simulink model "CORDIC_SAP"  (R2021a)
settings: Solver=VariableStepAuto  StartTime=0.0  StopTime=10.0  RelTol=1e-3
undefined symbols (not defined in the file or in its folder): AXI4, Lite
libraries: hdlBasic x278, xbsIndex_r4 x1
(part 1 of 3)
settings Model: Creator=jz118  LastModifiedBy=jz118

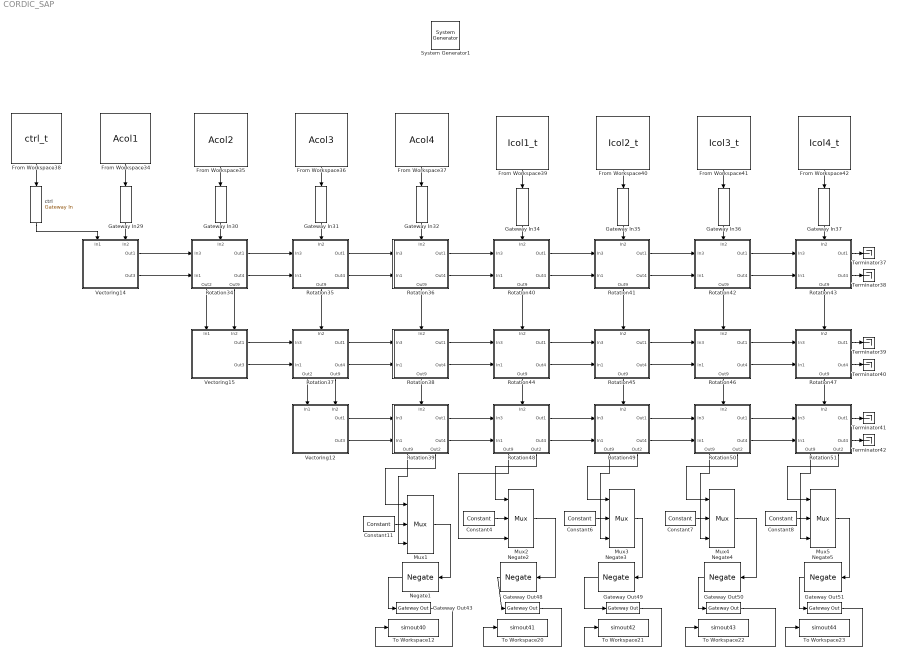
== system CORDIC_SAP ==
  " System Generator1" : xbsIndex_r4/ System Generator  Tag=genX  xilinxfamily=zynq  part=xc7z020  speed=-1  package=clg484  synthesis_tool=Vivado  clock_wrapper=Clock Enables  directory=./netlistAA  proj_type=Vivado  Synth_file=Vivado Synthesis Defaults  Impl_file=Vivado Implementation Defaults  testbench=off  simulink_period=1  sysclk_period=10  dcm_input_clock_period=10  incr_netlist=off  trim_vbits=Everywhere in SubSystem  dbl_ovrd=According to Block Masks  core_generation=According to Block Masks  run_coregen=off  deprecated_control=off  eval_field=0  block_type=sysgen
  Constant{4,6..8,11} (5 alike) : hdlBasic/Constant  const=0  gui_display_data_type=Fixed-point  arith_type=Signed (2's comp)  n_bits=16  bin_pt=13  preci_type=Single  exp_width=8  frac_width=24  explicit_period=off  period=1  XmcBlockStatus=1  maskContainerNames=tabcontainer1  block_type=constant  block_config=sysgen:Constant_config
  From Workspace34 : FromWorkspace  VariableName=Acol1
  From Workspace35 : FromWorkspace  VariableName=Acol2
  From Workspace36 : FromWorkspace  VariableName=Acol3
  From Workspace37 : FromWorkspace  VariableName=Acol4
  From Workspace38 : FromWorkspace  VariableName=ctrl_t
  From Workspace39 : FromWorkspace  VariableName=Icol1_t
  From Workspace40 : FromWorkspace  VariableName=Icol2_t
  From Workspace41 : FromWorkspace  VariableName=Icol3_t
  From Workspace42 : FromWorkspace  VariableName=Icol4_t
  Gateway In29 : hdlBasic/Gateway In  gui_display_data_type=Fixed-point  arith_type=Signed (2's comp)  n_bits=16  bin_pt=13  preci_type=Single  exp_width=8  frac_width=24  rows=1  columns=1  quantization="Round  (unbiased: +/- Inf)"  overflow=Saturate  period=1  UseAsADC=off  ADCChannel='1'  interface=AXI4-Lite  automatic_assignment=on  address_offset=hex2dec('00')  intf_name=''  intf_description='Acol1'  default_value=0  timing_constraint=None  locs_specified=off  LOCs={}  io_standard={}  inherit_from_input=off  hdl_port=on  XmcBlockStatus=1  maskContainerNames=group4  block_type=gatewayin  block_config=sysgen:gateway_in_config  block_width_w=590  block_height_w=620  block_width=640  block_height=850
  Gateway In30 : hdlBasic/Gateway In  gui_display_data_type=Fixed-point  arith_type=Signed (2's comp)  n_bits=16  bin_pt=13  preci_type=Single  exp_width=8  frac_width=24  rows=1  columns=1  quantization="Round  (unbiased: +/- Inf)"  overflow=Saturate  period=1  UseAsADC=off  ADCChannel='1'  interface=AXI4-Lite  automatic_assignment=on  address_offset=hex2dec('00')  intf_name=''  intf_description='Acol2'  default_value=0  timing_constraint=None  locs_specified=off  LOCs={}  io_standard={}  inherit_from_input=off  hdl_port=on  XmcBlockStatus=1  maskContainerNames=group4  block_type=gatewayin  block_config=sysgen:gateway_in_config  block_width_w=590  block_height_w=620  block_width=640  block_height=850
  Gateway In31 : hdlBasic/Gateway In  gui_display_data_type=Fixed-point  arith_type=Signed (2's comp)  n_bits=16  bin_pt=13  preci_type=Single  exp_width=8  frac_width=24  rows=1  columns=1  quantization="Round  (unbiased: +/- Inf)"  overflow=Saturate  period=1  UseAsADC=off  ADCChannel='1'  interface=AXI4-Lite  automatic_assignment=on  address_offset=hex2dec('00')  intf_name=''  intf_description='Acol3'  default_value=0  timing_constraint=None  locs_specified=off  LOCs={}  io_standard={}  inherit_from_input=off  hdl_port=on  XmcBlockStatus=1  maskContainerNames=group4  block_type=gatewayin  block_config=sysgen:gateway_in_config  block_width_w=590  block_height_w=620  block_width=640  block_height=850
  Gateway In32 : hdlBasic/Gateway In  gui_display_data_type=Fixed-point  arith_type=Signed (2's comp)  n_bits=16  bin_pt=13  preci_type=Single  exp_width=8  frac_width=24  rows=1  columns=1  quantization="Round  (unbiased: +/- Inf)"  overflow=Saturate  period=1  UseAsADC=off  ADCChannel='1'  interface=AXI4-Lite  automatic_assignment=on  address_offset=hex2dec('00')  intf_name=''  intf_description='Acol4'  default_value=0  timing_constraint=None  locs_specified=off  LOCs={}  io_standard={}  inherit_from_input=off  hdl_port=on  XmcBlockStatus=1  maskContainerNames=group4  block_type=gatewayin  block_config=sysgen:gateway_in_config  block_width_w=590  block_height_w=620  block_width=640  block_height=850
  Gateway In34 : hdlBasic/Gateway In  gui_display_data_type=Fixed-point  arith_type=Signed (2's comp)  n_bits=16  bin_pt=13  preci_type=Single  exp_width=8  frac_width=24  rows=1  columns=1  quantization="Round  (unbiased: +/- Inf)"  overflow=Saturate  period=1  UseAsADC=off  ADCChannel='1'  interface=AXI4-Lite  automatic_assignment=on  address_offset=hex2dec('00')  intf_name=''  intf_description='Icol1_t'  default_value=0  timing_constraint=None  locs_specified=off  LOCs={}  io_standard={}  inherit_from_input=off  hdl_port=on  XmcBlockStatus=1  maskContainerNames=group4  block_type=gatewayin  block_config=sysgen:gateway_in_config  block_width_w=590  block_height_w=620  block_width=640  block_height=850
  Gateway In35 : hdlBasic/Gateway In  gui_display_data_type=Fixed-point  arith_type=Signed (2's comp)  n_bits=16  bin_pt=13  preci_type=Single  exp_width=8  frac_width=24  rows=1  columns=1  quantization="Round  (unbiased: +/- Inf)"  overflow=Saturate  period=1  UseAsADC=off  ADCChannel='1'  interface=AXI4-Lite  automatic_assignment=on  address_offset=hex2dec('00')  intf_name=''  intf_description='Icol2_t'  default_value=0  timing_constraint=None  locs_specified=off  LOCs={}  io_standard={}  inherit_from_input=off  hdl_port=on  XmcBlockStatus=1  maskContainerNames=group4  block_type=gatewayin  block_config=sysgen:gateway_in_config  block_width_w=590  block_height_w=620  block_width=640  block_height=850
  Gateway In36 : hdlBasic/Gateway In  gui_display_data_type=Fixed-point  arith_type=Signed (2's comp)  n_bits=16  bin_pt=13  preci_type=Single  exp_width=8  frac_width=24  rows=1  columns=1  quantization="Round  (unbiased: +/- Inf)"  overflow=Saturate  period=1  UseAsADC=off  ADCChannel='1'  interface=AXI4-Lite  automatic_assignment=on  address_offset=hex2dec('00')  intf_name=''  intf_description='Icol3_t'  default_value=0  timing_constraint=None  locs_specified=off  LOCs={}  io_standard={}  inherit_from_input=off  hdl_port=on  XmcBlockStatus=1  maskContainerNames=group4  block_type=gatewayin  block_config=sysgen:gateway_in_config  block_width_w=590  block_height_w=620  block_width=640  block_height=850
  Gateway In37 : hdlBasic/Gateway In  gui_display_data_type=Fixed-point  arith_type=Signed (2's comp)  n_bits=16  bin_pt=13  preci_type=Single  exp_width=8  frac_width=24  rows=1  columns=1  quantization="Round  (unbiased: +/- Inf)"  overflow=Saturate  period=1  UseAsADC=off  ADCChannel='1'  interface=AXI4-Lite  automatic_assignment=on  address_offset=hex2dec('00')  intf_name=''  intf_description='Icol4_t'  default_value=0  timing_constraint=None  locs_specified=off  LOCs={}  io_standard={}  inherit_from_input=off  hdl_port=on  XmcBlockStatus=1  maskContainerNames=group4  block_type=gatewayin  block_config=sysgen:gateway_in_config  block_width_w=590  block_height_w=620  block_width=640  block_height=850
  Gateway Out43 : hdlBasic/Gateway Out  inherit_from_input=off  hdl_port=on  rows=1  columns=1  UseAsDAC=off  DACChannel='1'  interface=AXI4-Lite  automatic_assignment=on  address_offset=hex2dec('00')  intf_name=''  intf_description='R_4_4'  timing_constraint=None  locs_specified=off  LOCs={}  io_standard={}  XmcBlockStatus=1  maskContainerNames=group4  block_type=gatewayout  block_config=sysgen:gateway_out_config  block_width_w=590  block_height_w=620  block_width=620  block_height=750
  Gateway Out48 : hdlBasic/Gateway Out  inherit_from_input=off  hdl_port=on  rows=1  columns=1  UseAsDAC=off  DACChannel='1'  interface=AXI4-Lite  automatic_assignment=on  address_offset=hex2dec('00')  intf_name=''  intf_description='Q_4_1'  timing_constraint=None  locs_specified=off  LOCs={}  io_standard={}  XmcBlockStatus=1  maskContainerNames=group4  block_type=gatewayout  block_config=sysgen:gateway_out_config  block_width_w=590  block_height_w=620  block_width=620  block_height=750
  Gateway Out49 : hdlBasic/Gateway Out  inherit_from_input=off  hdl_port=on  rows=1  columns=1  UseAsDAC=off  DACChannel='1'  interface=AXI4-Lite  automatic_assignment=on  address_offset=hex2dec('00')  intf_name=''  intf_description='Q_4_2'  timing_constraint=None  locs_specified=off  LOCs={}  io_standard={}  XmcBlockStatus=1  maskContainerNames=group4  block_type=gatewayout  block_config=sysgen:gateway_out_config  block_width_w=590  block_height_w=620  block_width=620  block_height=750
  Gateway Out50 : hdlBasic/Gateway Out  inherit_from_input=off  hdl_port=on  rows=1  columns=1  UseAsDAC=off  DACChannel='1'  interface=AXI4-Lite  automatic_assignment=on  address_offset=hex2dec('00')  intf_name=''  intf_description='Q_4_3'  timing_constraint=None  locs_specified=off  LOCs={}  io_standard={}  XmcBlockStatus=1  maskContainerNames=group4  block_type=gatewayout  block_config=sysgen:gateway_out_config  block_width_w=590  block_height_w=620  block_width=620  block_height=750
  Gateway Out51 : hdlBasic/Gateway Out  inherit_from_input=off  hdl_port=on  rows=1  columns=1  UseAsDAC=off  DACChannel='1'  interface=AXI4-Lite  automatic_assignment=on  address_offset=hex2dec('00')  intf_name=''  intf_description='Q_4_4'  timing_constraint=None  locs_specified=off  LOCs={}  io_standard={}  XmcBlockStatus=1  maskContainerNames=group4  block_type=gatewayout  block_config=sysgen:gateway_out_config  block_width_w=590  block_height_w=620  block_width=620  block_height=750
  Mux{1..5} (5 alike) : hdlBasic/Mux  inputs=2  en=off  latency=1  precision=Full  arith_type=Unsigned  n_bits=16  bin_pt=14  quantization=Truncate  overflow=Wrap  XmcBlockStatus=1  maskContainerNames=tabcontainer1  block_type=mux  block_config=sysgen:Mux_config
  Negate{1..5} (5 alike) : hdlBasic/Negate  precision=Full  arith_type=Unsigned  n_bits=16  bin_pt=14  quantization=Truncate  overflow=Wrap  en=off  latency=0  XmcBlockStatus=1  maskContainerNames=tabcontainer1  block_type=negate  block_config=sysgen:Negate_config
  Rotation34 : Subsystem
      settings: PortSchema="{\"entries\":[{\"content\":{\"sides\":[{\"content\":{\"connectorIds\":[\"In1\",\"In2\"]},\"type\":\"ConnectorPlacement.EquallySpacedRectSide\",\"uuid\":\"b989bfd3-647b-468d-a24b-67c5817c2fb9\"},{\"content\":{\"connectorIds\":[\"Out1\",\"Out2\"],\"side\":\"RIGHT\"},\"type\":\"ConnectorPlacement.EquallySpacedRectSide\",\"uuid\":\"15839450-c6b9-4b4c-b490-793a0225ad70\"},{\"content\":{\"connectorIds\":[\"In3\"],\"side\":\"TOP\"},\"type\":\"ConnectorPlacement.EquallySpacedRectSide\",\"uuid\":\"69a0ff69-1754-49ce-bc12-3d58954b90b5\"},{\"content\":{\"connectorIds\":[\"Out3\",\"Out4\"],\"side\":\"BOTTOM\"},\"type\":\"ConnectorPlacement.EquallySpacedRectSide\",\"uuid\":\"c7c95c77-bae3-47b7-a54f-9afc9f4e7b60\"}]},\"type\":\"ConnectorPlacement.EquallySpacedConnector\",\"uuid\":\"47487c21-2009-4dc3-9515-f1b42d882620\"}],\"packageUris\":[\"http://schema.mathworks.com/mf0/Connector/R2020b\"],\"version\":\"1.0\"}"
  Rotation35 : Subsystem
      settings: PortSchema="{\"entries\":[{\"content\":{\"sides\":[{\"content\":{\"connectorIds\":[\"In1\",\"In2\"]},\"type\":\"ConnectorPlacement.EquallySpacedRectSide\",\"uuid\":\"b989bfd3-647b-468d-a24b-67c5817c2fb9\"},{\"content\":{\"connectorIds\":[\"Out1\",\"Out2\"],\"side\":\"RIGHT\"},\"type\":\"ConnectorPlacement.EquallySpacedRectSide\",\"uuid\":\"15839450-c6b9-4b4c-b490-793a0225ad70\"},{\"content\":{\"connectorIds\":[\"In3\"],\"side\":\"TOP\"},\"type\":\"ConnectorPlacement.EquallySpacedRectSide\",\"uuid\":\"69a0ff69-1754-49ce-bc12-3d58954b90b5\"},{\"content\":{\"connectorIds\":[\"Out3\"],\"side\":\"BOTTOM\"},\"type\":\"ConnectorPlacement.EquallySpacedRectSide\",\"uuid\":\"c7c95c77-bae3-47b7-a54f-9afc9f4e7b60\"}]},\"type\":\"ConnectorPlacement.EquallySpacedConnector\",\"uuid\":\"47487c21-2009-4dc3-9515-f1b42d882620\"}],\"packageUris\":[\"http://schema.mathworks.com/mf0/Connector/R2020b\"],\"version\":\"1.0\"}"
  Rotation36 : Subsystem
      settings: PortSchema="{\"entries\":[{\"content\":{\"sides\":[{\"content\":{\"connectorIds\":[\"In1\",\"In2\"]},\"type\":\"ConnectorPlacement.EquallySpacedRectSide\",\"uuid\":\"b989bfd3-647b-468d-a24b-67c5817c2fb9\"},{\"content\":{\"connectorIds\":[\"Out1\",\"Out2\"],\"side\":\"RIGHT\"},\"type\":\"ConnectorPlacement.EquallySpacedRectSide\",\"uuid\":\"15839450-c6b9-4b4c-b490-793a0225ad70\"},{\"content\":{\"connectorIds\":[\"In3\"],\"side\":\"TOP\"},\"type\":\"ConnectorPlacement.EquallySpacedRectSide\",\"uuid\":\"69a0ff69-1754-49ce-bc12-3d58954b90b5\"},{\"content\":{\"connectorIds\":[\"Out3\"],\"side\":\"BOTTOM\"},\"type\":\"ConnectorPlacement.EquallySpacedRectSide\",\"uuid\":\"c7c95c77-bae3-47b7-a54f-9afc9f4e7b60\"}]},\"type\":\"ConnectorPlacement.EquallySpacedConnector\",\"uuid\":\"47487c21-2009-4dc3-9515-f1b42d882620\"}],\"packageUris\":[\"http://schema.mathworks.com/mf0/Connector/R2020b\"],\"version\":\"1.0\"}"
  Rotation37 : Subsystem
      settings: PortSchema="{\"entries\":[{\"content\":{\"sides\":[{\"content\":{\"connectorIds\":[\"In1\",\"In2\"]},\"type\":\"ConnectorPlacement.EquallySpacedRectSide\",\"uuid\":\"b989bfd3-647b-468d-a24b-67c5817c2fb9\"},{\"content\":{\"connectorIds\":[\"Out1\",\"Out2\"],\"side\":\"RIGHT\"},\"type\":\"ConnectorPlacement.EquallySpacedRectSide\",\"uuid\":\"15839450-c6b9-4b4c-b490-793a0225ad70\"},{\"content\":{\"connectorIds\":[\"In3\"],\"side\":\"TOP\"},\"type\":\"ConnectorPlacement.EquallySpacedRectSide\",\"uuid\":\"69a0ff69-1754-49ce-bc12-3d58954b90b5\"},{\"content\":{\"connectorIds\":[\"Out3\",\"Out4\"],\"side\":\"BOTTOM\"},\"type\":\"ConnectorPlacement.EquallySpacedRectSide\",\"uuid\":\"c7c95c77-bae3-47b7-a54f-9afc9f4e7b60\"}]},\"type\":\"ConnectorPlacement.EquallySpacedConnector\",\"uuid\":\"47487c21-2009-4dc3-9515-f1b42d882620\"}],\"packageUris\":[\"http://schema.mathworks.com/mf0/Connector/R2020b\"],\"version\":\"1.0\"}"
  Rotation38 : Subsystem
      settings: PortSchema="{\"entries\":[{\"content\":{\"sides\":[{\"content\":{\"connectorIds\":[\"In1\",\"In2\"]},\"type\":\"ConnectorPlacement.EquallySpacedRectSide\",\"uuid\":\"b989bfd3-647b-468d-a24b-67c5817c2fb9\"},{\"content\":{\"connectorIds\":[\"Out1\",\"Out2\"],\"side\":\"RIGHT\"},\"type\":\"ConnectorPlacement.EquallySpacedRectSide\",\"uuid\":\"15839450-c6b9-4b4c-b490-793a0225ad70\"},{\"content\":{\"connectorIds\":[\"In3\"],\"side\":\"TOP\"},\"type\":\"ConnectorPlacement.EquallySpacedRectSide\",\"uuid\":\"69a0ff69-1754-49ce-bc12-3d58954b90b5\"},{\"content\":{\"connectorIds\":[\"Out3\"],\"side\":\"BOTTOM\"},\"type\":\"ConnectorPlacement.EquallySpacedRectSide\",\"uuid\":\"c7c95c77-bae3-47b7-a54f-9afc9f4e7b60\"}]},\"type\":\"ConnectorPlacement.EquallySpacedConnector\",\"uuid\":\"47487c21-2009-4dc3-9515-f1b42d882620\"}],\"packageUris\":[\"http://schema.mathworks.com/mf0/Connector/R2020b\"],\"version\":\"1.0\"}"
  Rotation39 : Subsystem
      settings: PortSchema="{\"entries\":[{\"content\":{\"sides\":[{\"content\":{\"connectorIds\":[\"In1\",\"In2\"]},\"type\":\"ConnectorPlacement.EquallySpacedRectSide\",\"uuid\":\"b989bfd3-647b-468d-a24b-67c5817c2fb9\"},{\"content\":{\"connectorIds\":[\"Out1\",\"Out2\"],\"side\":\"RIGHT\"},\"type\":\"ConnectorPlacement.EquallySpacedRectSide\",\"uuid\":\"15839450-c6b9-4b4c-b490-793a0225ad70\"},{\"content\":{\"connectorIds\":[\"In3\"],\"side\":\"TOP\"},\"type\":\"ConnectorPlacement.EquallySpacedRectSide\",\"uuid\":\"69a0ff69-1754-49ce-bc12-3d58954b90b5\"},{\"content\":{\"connectorIds\":[\"Out3\",\"Out4\"],\"side\":\"BOTTOM\"},\"type\":\"ConnectorPlacement.EquallySpacedRectSide\",\"uuid\":\"c7c95c77-bae3-47b7-a54f-9afc9f4e7b60\"}]},\"type\":\"ConnectorPlacement.EquallySpacedConnector\",\"uuid\":\"47487c21-2009-4dc3-9515-f1b42d882620\"}],\"packageUris\":[\"http://schema.mathworks.com/mf0/Connector/R2020b\"],\"version\":\"1.0\"}"
  Rotation40 : Subsystem
      settings: PortSchema="{\"entries\":[{\"content\":{\"sides\":[{\"content\":{\"connectorIds\":[\"In1\",\"In2\"]},\"type\":\"ConnectorPlacement.EquallySpacedRectSide\",\"uuid\":\"b989bfd3-647b-468d-a24b-67c5817c2fb9\"},{\"content\":{\"connectorIds\":[\"Out1\",\"Out2\"],\"side\":\"RIGHT\"},\"type\":\"ConnectorPlacement.EquallySpacedRectSide\",\"uuid\":\"15839450-c6b9-4b4c-b490-793a0225ad70\"},{\"content\":{\"connectorIds\":[\"In3\"],\"side\":\"TOP\"},\"type\":\"ConnectorPlacement.EquallySpacedRectSide\",\"uuid\":\"69a0ff69-1754-49ce-bc12-3d58954b90b5\"},{\"content\":{\"connectorIds\":[\"Out3\"],\"side\":\"BOTTOM\"},\"type\":\"ConnectorPlacement.EquallySpacedRectSide\",\"uuid\":\"c7c95c77-bae3-47b7-a54f-9afc9f4e7b60\"}]},\"type\":\"ConnectorPlacement.EquallySpacedConnector\",\"uuid\":\"47487c21-2009-4dc3-9515-f1b42d882620\"}],\"packageUris\":[\"http://schema.mathworks.com/mf0/Connector/R2020b\"],\"version\":\"1.0\"}"
  Rotation41 : Subsystem
      settings: PortSchema="{\"entries\":[{\"content\":{\"sides\":[{\"content\":{\"connectorIds\":[\"In1\",\"In2\"]},\"type\":\"ConnectorPlacement.EquallySpacedRectSide\",\"uuid\":\"b989bfd3-647b-468d-a24b-67c5817c2fb9\"},{\"content\":{\"connectorIds\":[\"Out1\",\"Out2\"],\"side\":\"RIGHT\"},\"type\":\"ConnectorPlacement.EquallySpacedRectSide\",\"uuid\":\"15839450-c6b9-4b4c-b490-793a0225ad70\"},{\"content\":{\"connectorIds\":[\"In3\"],\"side\":\"TOP\"},\"type\":\"ConnectorPlacement.EquallySpacedRectSide\",\"uuid\":\"69a0ff69-1754-49ce-bc12-3d58954b90b5\"},{\"content\":{\"connectorIds\":[\"Out3\"],\"side\":\"BOTTOM\"},\"type\":\"ConnectorPlacement.EquallySpacedRectSide\",\"uuid\":\"c7c95c77-bae3-47b7-a54f-9afc9f4e7b60\"}]},\"type\":\"ConnectorPlacement.EquallySpacedConnector\",\"uuid\":\"47487c21-2009-4dc3-9515-f1b42d882620\"}],\"packageUris\":[\"http://schema.mathworks.com/mf0/Connector/R2020b\"],\"version\":\"1.0\"}"
  Rotation42 : Subsystem
      settings: PortSchema="{\"entries\":[{\"content\":{\"sides\":[{\"content\":{\"connectorIds\":[\"In1\",\"In2\"]},\"type\":\"ConnectorPlacement.EquallySpacedRectSide\",\"uuid\":\"b989bfd3-647b-468d-a24b-67c5817c2fb9\"},{\"content\":{\"connectorIds\":[\"Out1\",\"Out2\"],\"side\":\"RIGHT\"},\"type\":\"ConnectorPlacement.EquallySpacedRectSide\",\"uuid\":\"15839450-c6b9-4b4c-b490-793a0225ad70\"},{\"content\":{\"connectorIds\":[\"In3\"],\"side\":\"TOP\"},\"type\":\"ConnectorPlacement.EquallySpacedRectSide\",\"uuid\":\"69a0ff69-1754-49ce-bc12-3d58954b90b5\"},{\"content\":{\"connectorIds\":[\"Out3\"],\"side\":\"BOTTOM\"},\"type\":\"ConnectorPlacement.EquallySpacedRectSide\",\"uuid\":\"c7c95c77-bae3-47b7-a54f-9afc9f4e7b60\"}]},\"type\":\"ConnectorPlacement.EquallySpacedConnector\",\"uuid\":\"47487c21-2009-4dc3-9515-f1b42d882620\"}],\"packageUris\":[\"http://schema.mathworks.com/mf0/Connector/R2020b\"],\"version\":\"1.0\"}"
  Rotation43 : Subsystem
      settings: PortSchema="{\"entries\":[{\"content\":{\"sides\":[{\"content\":{\"connectorIds\":[\"In1\",\"In2\"]},\"type\":\"ConnectorPlacement.EquallySpacedRectSide\",\"uuid\":\"b989bfd3-647b-468d-a24b-67c5817c2fb9\"},{\"content\":{\"connectorIds\":[\"Out1\",\"Out2\"],\"side\":\"RIGHT\"},\"type\":\"ConnectorPlacement.EquallySpacedRectSide\",\"uuid\":\"15839450-c6b9-4b4c-b490-793a0225ad70\"},{\"content\":{\"connectorIds\":[\"In3\"],\"side\":\"TOP\"},\"type\":\"ConnectorPlacement.EquallySpacedRectSide\",\"uuid\":\"69a0ff69-1754-49ce-bc12-3d58954b90b5\"},{\"content\":{\"connectorIds\":[\"Out3\"],\"side\":\"BOTTOM\"},\"type\":\"ConnectorPlacement.EquallySpacedRectSide\",\"uuid\":\"c7c95c77-bae3-47b7-a54f-9afc9f4e7b60\"}]},\"type\":\"ConnectorPlacement.EquallySpacedConnector\",\"uuid\":\"47487c21-2009-4dc3-9515-f1b42d882620\"}],\"packageUris\":[\"http://schema.mathworks.com/mf0/Connector/R2020b\"],\"version\":\"1.0\"}"
  Rotation44 : Subsystem
      settings: PortSchema="{\"entries\":[{\"content\":{\"sides\":[{\"content\":{\"connectorIds\":[\"In1\",\"In2\"]},\"type\":\"ConnectorPlacement.EquallySpacedRectSide\",\"uuid\":\"b989bfd3-647b-468d-a24b-67c5817c2fb9\"},{\"content\":{\"connectorIds\":[\"Out1\",\"Out2\"],\"side\":\"RIGHT\"},\"type\":\"ConnectorPlacement.EquallySpacedRectSide\",\"uuid\":\"15839450-c6b9-4b4c-b490-793a0225ad70\"},{\"content\":{\"connectorIds\":[\"In3\"],\"side\":\"TOP\"},\"type\":\"ConnectorPlacement.EquallySpacedRectSide\",\"uuid\":\"69a0ff69-1754-49ce-bc12-3d58954b90b5\"},{\"content\":{\"connectorIds\":[\"Out3\"],\"side\":\"BOTTOM\"},\"type\":\"ConnectorPlacement.EquallySpacedRectSide\",\"uuid\":\"c7c95c77-bae3-47b7-a54f-9afc9f4e7b60\"}]},\"type\":\"ConnectorPlacement.EquallySpacedConnector\",\"uuid\":\"47487c21-2009-4dc3-9515-f1b42d882620\"}],\"packageUris\":[\"http://schema.mathworks.com/mf0/Connector/R2020b\"],\"version\":\"1.0\"}"
  Rotation45 : Subsystem
      settings: PortSchema="{\"entries\":[{\"content\":{\"sides\":[{\"content\":{\"connectorIds\":[\"In1\",\"In2\"]},\"type\":\"ConnectorPlacement.EquallySpacedRectSide\",\"uuid\":\"b989bfd3-647b-468d-a24b-67c5817c2fb9\"},{\"content\":{\"connectorIds\":[\"Out1\",\"Out2\"],\"side\":\"RIGHT\"},\"type\":\"ConnectorPlacement.EquallySpacedRectSide\",\"uuid\":\"15839450-c6b9-4b4c-b490-793a0225ad70\"},{\"content\":{\"connectorIds\":[\"In3\"],\"side\":\"TOP\"},\"type\":\"ConnectorPlacement.EquallySpacedRectSide\",\"uuid\":\"69a0ff69-1754-49ce-bc12-3d58954b90b5\"},{\"content\":{\"connectorIds\":[\"Out3\"],\"side\":\"BOTTOM\"},\"type\":\"ConnectorPlacement.EquallySpacedRectSide\",\"uuid\":\"c7c95c77-bae3-47b7-a54f-9afc9f4e7b60\"}]},\"type\":\"ConnectorPlacement.EquallySpacedConnector\",\"uuid\":\"47487c21-2009-4dc3-9515-f1b42d882620\"}],\"packageUris\":[\"http://schema.mathworks.com/mf0/Connector/R2020b\"],\"version\":\"1.0\"}"
  Rotation46 : Subsystem
      settings: PortSchema="{\"entries\":[{\"content\":{\"sides\":[{\"content\":{\"connectorIds\":[\"In1\",\"In2\"]},\"type\":\"ConnectorPlacement.EquallySpacedRectSide\",\"uuid\":\"b989bfd3-647b-468d-a24b-67c5817c2fb9\"},{\"content\":{\"connectorIds\":[\"Out1\",\"Out2\"],\"side\":\"RIGHT\"},\"type\":\"ConnectorPlacement.EquallySpacedRectSide\",\"uuid\":\"15839450-c6b9-4b4c-b490-793a0225ad70\"},{\"content\":{\"connectorIds\":[\"In3\"],\"side\":\"TOP\"},\"type\":\"ConnectorPlacement.EquallySpacedRectSide\",\"uuid\":\"69a0ff69-1754-49ce-bc12-3d58954b90b5\"},{\"content\":{\"connectorIds\":[\"Out3\"],\"side\":\"BOTTOM\"},\"type\":\"ConnectorPlacement.EquallySpacedRectSide\",\"uuid\":\"c7c95c77-bae3-47b7-a54f-9afc9f4e7b60\"}]},\"type\":\"ConnectorPlacement.EquallySpacedConnector\",\"uuid\":\"47487c21-2009-4dc3-9515-f1b42d882620\"}],\"packageUris\":[\"http://schema.mathworks.com/mf0/Connector/R2020b\"],\"version\":\"1.0\"}"
  Rotation47 : Subsystem
      settings: PortSchema="{\"entries\":[{\"content\":{\"sides\":[{\"content\":{\"connectorIds\":[\"In1\",\"In2\"]},\"type\":\"ConnectorPlacement.EquallySpacedRectSide\",\"uuid\":\"b989bfd3-647b-468d-a24b-67c5817c2fb9\"},{\"content\":{\"connectorIds\":[\"Out1\",\"Out2\"],\"side\":\"RIGHT\"},\"type\":\"ConnectorPlacement.EquallySpacedRectSide\",\"uuid\":\"15839450-c6b9-4b4c-b490-793a0225ad70\"},{\"content\":{\"connectorIds\":[\"In3\"],\"side\":\"TOP\"},\"type\":\"ConnectorPlacement.EquallySpacedRectSide\",\"uuid\":\"69a0ff69-1754-49ce-bc12-3d58954b90b5\"},{\"content\":{\"connectorIds\":[\"Out3\"],\"side\":\"BOTTOM\"},\"type\":\"ConnectorPlacement.EquallySpacedRectSide\",\"uuid\":\"c7c95c77-bae3-47b7-a54f-9afc9f4e7b60\"}]},\"type\":\"ConnectorPlacement.EquallySpacedConnector\",\"uuid\":\"47487c21-2009-4dc3-9515-f1b42d882620\"}],\"packageUris\":[\"http://schema.mathworks.com/mf0/Connector/R2020b\"],\"version\":\"1.0\"}"
  Rotation48 : Subsystem
      settings: PortSchema="{\"entries\":[{\"content\":{\"sides\":[{\"content\":{\"connectorIds\":[\"In1\",\"In2\"]},\"type\":\"ConnectorPlacement.EquallySpacedRectSide\",\"uuid\":\"b989bfd3-647b-468d-a24b-67c5817c2fb9\"},{\"content\":{\"connectorIds\":[\"Out1\",\"Out2\"],\"side\":\"RIGHT\"},\"type\":\"ConnectorPlacement.EquallySpacedRectSide\",\"uuid\":\"15839450-c6b9-4b4c-b490-793a0225ad70\"},{\"content\":{\"connectorIds\":[\"In3\"],\"side\":\"TOP\"},\"type\":\"ConnectorPlacement.EquallySpacedRectSide\",\"uuid\":\"69a0ff69-1754-49ce-bc12-3d58954b90b5\"},{\"content\":{\"connectorIds\":[\"Out3\",\"Out4\"],\"side\":\"BOTTOM\"},\"type\":\"ConnectorPlacement.EquallySpacedRectSide\",\"uuid\":\"c7c95c77-bae3-47b7-a54f-9afc9f4e7b60\"}]},\"type\":\"ConnectorPlacement.EquallySpacedConnector\",\"uuid\":\"47487c21-2009-4dc3-9515-f1b42d882620\"}],\"packageUris\":[\"http://schema.mathworks.com/mf0/Connector/R2020b\"],\"version\":\"1.0\"}"
  Rotation49 : Subsystem
      settings: PortSchema="{\"entries\":[{\"content\":{\"sides\":[{\"content\":{\"connectorIds\":[\"In1\",\"In2\"]},\"type\":\"ConnectorPlacement.EquallySpacedRectSide\",\"uuid\":\"b989bfd3-647b-468d-a24b-67c5817c2fb9\"},{\"content\":{\"connectorIds\":[\"Out1\",\"Out2\"],\"side\":\"RIGHT\"},\"type\":\"ConnectorPlacement.EquallySpacedRectSide\",\"uuid\":\"15839450-c6b9-4b4c-b490-793a0225ad70\"},{\"content\":{\"connectorIds\":[\"In3\"],\"side\":\"TOP\"},\"type\":\"ConnectorPlacement.EquallySpacedRectSide\",\"uuid\":\"69a0ff69-1754-49ce-bc12-3d58954b90b5\"},{\"content\":{\"connectorIds\":[\"Out3\",\"Out4\"],\"side\":\"BOTTOM\"},\"type\":\"ConnectorPlacement.EquallySpacedRectSide\",\"uuid\":\"c7c95c77-bae3-47b7-a54f-9afc9f4e7b60\"}]},\"type\":\"ConnectorPlacement.EquallySpacedConnector\",\"uuid\":\"47487c21-2009-4dc3-9515-f1b42d882620\"}],\"packageUris\":[\"http://schema.mathworks.com/mf0/Connector/R2020b\"],\"version\":\"1.0\"}"
  Rotation50 : Subsystem
      settings: PortSchema="{\"entries\":[{\"content\":{\"sides\":[{\"content\":{\"connectorIds\":[\"In1\",\"In2\"]},\"type\":\"ConnectorPlacement.EquallySpacedRectSide\",\"uuid\":\"b989bfd3-647b-468d-a24b-67c5817c2fb9\"},{\"content\":{\"connectorIds\":[\"Out1\",\"Out2\"],\"side\":\"RIGHT\"},\"type\":\"ConnectorPlacement.EquallySpacedRectSide\",\"uuid\":\"15839450-c6b9-4b4c-b490-793a0225ad70\"},{\"content\":{\"connectorIds\":[\"In3\"],\"side\":\"TOP\"},\"type\":\"ConnectorPlacement.EquallySpacedRectSide\",\"uuid\":\"69a0ff69-1754-49ce-bc12-3d58954b90b5\"},{\"content\":{\"connectorIds\":[\"Out3\",\"Out4\"],\"side\":\"BOTTOM\"},\"type\":\"ConnectorPlacement.EquallySpacedRectSide\",\"uuid\":\"c7c95c77-bae3-47b7-a54f-9afc9f4e7b60\"}]},\"type\":\"ConnectorPlacement.EquallySpacedConnector\",\"uuid\":\"47487c21-2009-4dc3-9515-f1b42d882620\"}],\"packageUris\":[\"http://schema.mathworks.com/mf0/Connector/R2020b\"],\"version\":\"1.0\"}"
  Rotation51 : Subsystem
      settings: PortSchema="{\"entries\":[{\"content\":{\"sides\":[{\"content\":{\"connectorIds\":[\"In1\",\"In2\"]},\"type\":\"ConnectorPlacement.EquallySpacedRectSide\",\"uuid\":\"b989bfd3-647b-468d-a24b-67c5817c2fb9\"},{\"content\":{\"connectorIds\":[\"Out1\",\"Out2\"],\"side\":\"RIGHT\"},\"type\":\"ConnectorPlacement.EquallySpacedRectSide\",\"uuid\":\"15839450-c6b9-4b4c-b490-793a0225ad70\"},{\"content\":{\"connectorIds\":[\"In3\"],\"side\":\"TOP\"},\"type\":\"ConnectorPlacement.EquallySpacedRectSide\",\"uuid\":\"69a0ff69-1754-49ce-bc12-3d58954b90b5\"},{\"content\":{\"connectorIds\":[\"Out3\",\"Out4\"],\"side\":\"BOTTOM\"},\"type\":\"ConnectorPlacement.EquallySpacedRectSide\",\"uuid\":\"c7c95c77-bae3-47b7-a54f-9afc9f4e7b60\"}]},\"type\":\"ConnectorPlacement.EquallySpacedConnector\",\"uuid\":\"47487c21-2009-4dc3-9515-f1b42d882620\"}],\"packageUris\":[\"http://schema.mathworks.com/mf0/Connector/R2020b\"],\"version\":\"1.0\"}"
  Terminator{37..42} (6 alike) : Terminator
  To Workspace12 : ToWorkspace  VariableName=simout40  SaveFormat=Timeseries  SampleTime=-1
  To Workspace20 : ToWorkspace  VariableName=simout41  SaveFormat=Timeseries  SampleTime=-1
  To Workspace21 : ToWorkspace  VariableName=simout42  SaveFormat=Timeseries  SampleTime=-1
  To Workspace22 : ToWorkspace  VariableName=simout43  SaveFormat=Timeseries  SampleTime=-1
  To Workspace23 : ToWorkspace  VariableName=simout44  SaveFormat=Timeseries  SampleTime=-1
  Vectoring12 : Subsystem
      settings: PortSchema="{\"entries\":[{\"content\":{\"sides\":[{\"content\":{\"connectorIds\":[]},\"type\":\"ConnectorPlacement.EquallySpacedRectSide\",\"uuid\":\"7f0919a1-928c-4229-a557-ae6b37c0e18a\"},{\"content\":{\"connectorIds\":[\"Out1\",\"Out2\"],\"side\":\"RIGHT\"},\"type\":\"ConnectorPlacement.EquallySpacedRectSide\",\"uuid\":\"c3dbff62-2cbb-49e5-a718-27c684f0604c\"},{\"content\":{\"connectorIds\":[\"In1\",\"In2\"],\"side\":\"TOP\"},\"type\":\"ConnectorPlacement.EquallySpacedRectSide\",\"uuid\":\"83a064d4-85ee-4dcc-804e-22587799da9e\"},{\"content\":{\"connectorIds\":[],\"side\":\"BOTTOM\"},\"type\":\"ConnectorPlacement.EquallySpacedRectSide\",\"uuid\":\"eea76909-33f2-4847-bfa0-f6ca22c12ff2\"}]},\"type\":\"ConnectorPlacement.EquallySpacedConnector\",\"uuid\":\"6d33be0e-4d36-4c84-a292-f5ef4e252a8e\"}],\"packageUris\":[\"http://schema.mathworks.com/mf0/Connector/R2020b\"],\"version\":\"1.0\"}"
  Vectoring14 : Subsystem
      settings: PortSchema="{\"entries\":[{\"content\":{\"sides\":[{\"content\":{\"connectorIds\":[]},\"type\":\"ConnectorPlacement.EquallySpacedRectSide\",\"uuid\":\"7f0919a1-928c-4229-a557-ae6b37c0e18a\"},{\"content\":{\"connectorIds\":[\"Out1\",\"Out2\"],\"side\":\"RIGHT\"},\"type\":\"ConnectorPlacement.EquallySpacedRectSide\",\"uuid\":\"c3dbff62-2cbb-49e5-a718-27c684f0604c\"},{\"content\":{\"connectorIds\":[\"In1\",\"In2\"],\"side\":\"TOP\"},\"type\":\"ConnectorPlacement.EquallySpacedRectSide\",\"uuid\":\"83a064d4-85ee-4dcc-804e-22587799da9e\"},{\"content\":{\"connectorIds\":[],\"side\":\"BOTTOM\"},\"type\":\"ConnectorPlacement.EquallySpacedRectSide\",\"uuid\":\"eea76909-33f2-4847-bfa0-f6ca22c12ff2\"}]},\"type\":\"ConnectorPlacement.EquallySpacedConnector\",\"uuid\":\"6d33be0e-4d36-4c84-a292-f5ef4e252a8e\"}],\"packageUris\":[\"http://schema.mathworks.com/mf0/Connector/R2020b\"],\"version\":\"1.0\"}"
  Vectoring15 : Subsystem
      settings: PortSchema="{\"entries\":[{\"content\":{\"sides\":[{\"content\":{\"connectorIds\":[]},\"type\":\"ConnectorPlacement.EquallySpacedRectSide\",\"uuid\":\"7f0919a1-928c-4229-a557-ae6b37c0e18a\"},{\"content\":{\"connectorIds\":[\"Out1\",\"Out2\"],\"side\":\"RIGHT\"},\"type\":\"ConnectorPlacement.EquallySpacedRectSide\",\"uuid\":\"c3dbff62-2cbb-49e5-a718-27c684f0604c\"},{\"content\":{\"connectorIds\":[\"In1\",\"In2\"],\"side\":\"TOP\"},\"type\":\"ConnectorPlacement.EquallySpacedRectSide\",\"uuid\":\"83a064d4-85ee-4dcc-804e-22587799da9e\"},{\"content\":{\"connectorIds\":[],\"side\":\"BOTTOM\"},\"type\":\"ConnectorPlacement.EquallySpacedRectSide\",\"uuid\":\"eea76909-33f2-4847-bfa0-f6ca22c12ff2\"}]},\"type\":\"ConnectorPlacement.EquallySpacedConnector\",\"uuid\":\"6d33be0e-4d36-4c84-a292-f5ef4e252a8e\"}],\"packageUris\":[\"http://schema.mathworks.com/mf0/Connector/R2020b\"],\"version\":\"1.0\"}"
  ctrl : hdlBasic/Gateway In  gui_display_data_type=Boolean  arith_type=Boolean  n_bits=16  bin_pt=13  preci_type=Single  exp_width=8  frac_width=24  rows=1  columns=1  quantization="Round  (unbiased: +/- Inf)"  overflow=Saturate  period=1  UseAsADC=off  ADCChannel='1'  interface=AXI4-Lite  automatic_assignment=on  address_offset=hex2dec('00')  intf_name=''  intf_description='ctrl_t'  default_value=0  timing_constraint=None  locs_specified=off  LOCs={}  io_standard={}  inherit_from_input=off  hdl_port=on  XmcBlockStatus=1  maskContainerNames=group4  block_type=gatewayin  block_config=sysgen:gateway_in_config  block_width_w=590  block_height_w=620  block_width=640  block_height=850
  wires:
  Rotation46/2(Out4) -> Rotation47/2(In1)
  From Workspace40/1 -> Gateway In35/1
  Rotation50/3(Out9) -> Mux4/3
  Negate4/1 -> Gateway Out50/1
  Rotation43/1(Out1) -> Terminator37/1
  Mux3/1 -> Negate3/1
  Vectoring12/1(Out1) -> Rotation39/1(In3)
  Rotation37/2(Out4) -> Rotation38/2(In1)
  Rotation39/3(Out9) -> Mux1/3
  From Workspace42/1 -> Gateway In37/1
  Gateway In30/1 -> Rotation34/3(In2)
  Rotation40/1(Out1) -> Rotation41/1(In3)
  Gateway In32/1 -> Rotation36/3(In2)
  Mux4/1 -> Negate4/1
  Rotation45/3(Out9) -> Rotation49/3(In2)
  Rotation51/3(Out9) -> Mux5/3
  From Workspace36/1 -> Gateway In31/1
  From Workspace39/1 -> Gateway In34/1
  Negate3/1 -> Gateway Out49/1
  Mux2/1 -> Negate2/1
  Rotation40/2(Out4) -> Rotation41/2(In1)
  Rotation35/3(Out9) -> Rotation37/3(In2)
  Rotation48/3(Out9) -> Mux2/3
  Rotation48/2(Out4) -> Rotation49/2(In1)
  Gateway Out48/1 -> To Workspace20/1
  Negate2/1 -> Gateway Out48/1
  Rotation42/2(Out4) -> Rotation43/2(In1)
  Gateway Out50/1 -> To Workspace22/1
  Negate5/1 -> Gateway Out51/1
  Rotation37/1(Out1) -> Rotation38/1(In3)
  Rotation49/3(Out9) -> Mux3/3
  Negate1/1 -> Gateway Out43/1
  Rotation36/1(Out1) -> Rotation40/1(In3)
  Constant6/1 -> Mux3/2
  Constant8/1 -> Mux5/2
  Gateway Out51/1 -> To Workspace23/1
  Gateway Out43/1 -> To Workspace12/1
  Constant7/1 -> Mux4/2
  Constant4/1 -> Mux2/2
  Rotation47/1(Out1) -> Terminator39/1
  ctrl/1 -> Vectoring14/1(In1)
  Rotation51/2(Out4) -> Terminator42/1
  Rotation51/1(Out1) -> Terminator41/1
  Rotation47/2(Out4) -> Terminator40/1
  Rotation43/2(Out4) -> Terminator38/1
  From Workspace34/1 -> Gateway In29/1
  Rotation45/2(Out4) -> Rotation46/2(In1)
  Vectoring15/2(Out3) -> Rotation37/2(In1)
  Rotation41/1(Out1) -> Rotation42/1(In3)
  Gateway In37/1 -> Rotation43/3(In2)
  Rotation39/2(Out4) -> Rotation48/2(In1)
  Rotation49/2(Out4) -> Rotation50/2(In1)
  Vectoring14/2(Out3) -> Rotation34/2(In1)
  Gateway In34/1 -> Rotation40/3(In2)
  Rotation50/1(Out1) -> Rotation51/1(In3)
  Rotation42/1(Out1) -> Rotation43/1(In3)
  Rotation47/3(Out9) -> Rotation51/3(In2)
  Rotation48/1(Out1) -> Rotation49/1(In3)
  From Workspace35/1 -> Gateway In30/1
  Rotation46/3(Out9) -> Rotation50/3(In2)
  Rotation49/1(Out1) -> Rotation50/1(In3)
  Rotation36/2(Out4) -> Rotation40/2(In1)
  Rotation43/3(Out9) -> Rotation47/3(In2)
  Rotation42/3(Out9) -> Rotation46/3(In2)
  Rotation46/1(Out1) -> Rotation47/1(In3)
  Rotation38/2(Out4) -> Rotation44/2(In1)
  Rotation38/1(Out1) -> Rotation44/1(In3)
  Gateway In36/1 -> Rotation42/3(In2)
  Rotation41/2(Out4) -> Rotation42/2(In1)
  Mux1/1 -> Negate1/1
  Rotation40/3(Out9) -> Rotation44/3(In2)
  From Workspace41/1 -> Gateway In36/1
  Rotation39/1(Out1) -> Rotation48/1(In3)
  Constant11/1 -> Mux1/2
  Rotation41/3(Out9) -> Rotation45/3(In2)
  Gateway In35/1 -> Rotation41/3(In2)
  Gateway Out49/1 -> To Workspace21/1
  Rotation45/1(Out1) -> Rotation46/1(In3)
  Rotation44/3(Out9) -> Rotation48/3(In2)
  Rotation36/3(Out9) -> Rotation38/3(In2)
  Rotation38/3(Out9) -> Rotation39/3(In2)
  Vectoring12/2(Out3) -> Rotation39/2(In1)
  Rotation37/3(Out2) -> Vectoring12/1(In1)
  Rotation34/3(Out2) -> Vectoring15/1(In1)
  Mux5/1 -> Negate5/1
  Rotation44/2(Out4) -> Rotation45/2(In1)
  Vectoring15/1(Out1) -> Rotation37/1(In3)
  Gateway In29/1 -> Vectoring14/2(In2)
  Vectoring14/1(Out1) -> Rotation34/1(In3)
  Rotation34/2(Out4) -> Rotation35/2(In1)
  Rotation34/1(Out1) -> Rotation35/1(In3)
  Rotation35/1(Out1) -> Rotation36/1(In3)
  Rotation37/4(Out9) -> Vectoring12/2(In2)
  Rotation50/2(Out4) -> Rotation51/2(In1)
  From Workspace37/1 -> Gateway In32/1
  Rotation34/4(Out9) -> Vectoring15/2(In2)
  Rotation44/1(Out1) -> Rotation45/1(In3)
  Rotation35/2(Out4) -> Rotation36/2(In1)
  Gateway In31/1 -> Rotation35/3(In2)
  From Workspace38/1 -> ctrl/1
  Rotation39/4(Out2) -> Mux1/1
  Rotation51/4(Out2) -> Mux5/1
  Rotation50/4(Out2) -> Mux4/1
  Rotation49/4(Out2) -> Mux3/1
  Rotation48/4(Out2) -> Mux2/1

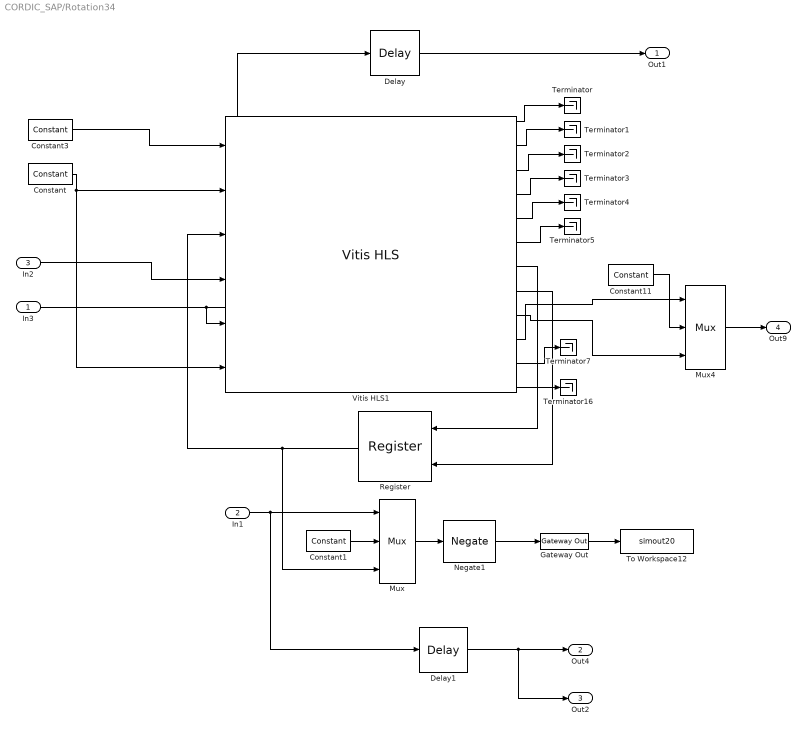
== system CORDIC_SAP/Rotation34 ==
  In3 : Inport
  In1 : Inport  Port=2
  In2 : Inport  Port=3
  Constant : hdlBasic/Constant  const=1.0  gui_display_data_type=Boolean  arith_type=Boolean  n_bits=16  bin_pt=14  preci_type=Single  exp_width=8  frac_width=24  explicit_period=off  period=1  XmcBlockStatus=1  maskContainerNames=tabcontainer1  block_type=constant  block_config=sysgen:Constant_config
  Constant1 : hdlBasic/Constant  const=0  gui_display_data_type=Fixed-point  arith_type=Signed (2's comp)  n_bits=16  bin_pt=13  preci_type=Single  exp_width=8  frac_width=24  explicit_period=off  period=1  XmcBlockStatus=1  maskContainerNames=tabcontainer1  block_type=constant  block_config=sysgen:Constant_config
  Constant11 : hdlBasic/Constant  const=0  gui_display_data_type=Fixed-point  arith_type=Signed (2's comp)  n_bits=16  bin_pt=13  preci_type=Single  exp_width=8  frac_width=24  explicit_period=off  period=1  XmcBlockStatus=1  maskContainerNames=tabcontainer1  block_type=constant  block_config=sysgen:Constant_config
  Constant3 : hdlBasic/Constant  const=0  gui_display_data_type=Boolean  arith_type=Boolean  n_bits=16  bin_pt=14  preci_type=Single  exp_width=8  frac_width=24  explicit_period=off  period=1  XmcBlockStatus=1  maskContainerNames=tabcontainer1  block_type=constant  block_config=sysgen:Constant_config
  Delay : hdlBasic/Delay  rst=off  en=off  latency=27  reg_retiming=off  XmcBlockStatus=1  maskContainerNames=group1  block_type=delay  block_config=sysgen:Delay_config
  Delay1 : hdlBasic/Delay  rst=off  en=off  latency=27  reg_retiming=off  XmcBlockStatus=1  maskContainerNames=group1  block_type=delay  block_config=sysgen:Delay_config
  Gateway Out : hdlBasic/Gateway Out  inherit_from_input=off  hdl_port=on  rows=1  columns=1  UseAsDAC=off  DACChannel='1'  interface=AXI4-Lite  automatic_assignment=on  address_offset=hex2dec('00')  intf_name=''  intf_description='R_1_2'  timing_constraint=None  locs_specified=off  LOCs={}  io_standard={}  XmcBlockStatus=1  maskContainerNames=group4  block_type=gatewayout  block_config=sysgen:gateway_out_config  block_width_w=590  block_height_w=620  block_width=620  block_height=750
  Mux : hdlBasic/Mux  inputs=2  en=off  latency=1  precision=Full  arith_type=Unsigned  n_bits=16  bin_pt=14  quantization=Truncate  overflow=Wrap  XmcBlockStatus=1  maskContainerNames=tabcontainer1  block_type=mux  block_config=sysgen:Mux_config
  Mux4 : hdlBasic/Mux  inputs=2  en=off  latency=1  precision=Full  arith_type=Unsigned  n_bits=16  bin_pt=14  quantization=Truncate  overflow=Wrap  XmcBlockStatus=1  maskContainerNames=tabcontainer1  block_type=mux  block_config=sysgen:Mux_config
  Negate1 : hdlBasic/Negate  precision=Full  arith_type=Unsigned  n_bits=16  bin_pt=14  quantization=Truncate  overflow=Wrap  en=off  latency=0  XmcBlockStatus=1  maskContainerNames=tabcontainer1  block_type=negate  block_config=sysgen:Negate_config
  Register : hdlBasic/Register  init=0  rst=off  en=on  XmcBlockStatus=1  maskContainerNames=tabcontainer1  block_type=register  block_config=sysgen:Register_config
  Terminator{,1..5,7,16} (8 alike) : Terminator
  To Workspace12 : ToWorkspace  VariableName=simout20  SaveFormat=Timeseries  SampleTime=-1
  Vitis HLS1 : hdlBasic/Vitis HLS  anytable='C:\ELEC522\jz118\HLS\cordic\solution1'  fast_sim=off  display_datatype=off  rate_propagation_method=Simulink system period  model_file_path=''  latency=1  block_type=vitis_hls
      settings: infoedit=This block allows including C,C++ and SystemC source files in System Generator for DSP designs.
  Out1 : Outport
  Out4 : Outport  Port=2
  Out2 : Outport  Port=3
  Out9 : Outport  Port=4
  wires:
  In2/1 -> Vitis HLS1/4
  In3/1 -> Delay/1, Vitis HLS1/5
  Delay/1 -> Out1/1
  Constant/1 -> Vitis HLS1/2, Vitis HLS1/6
  Constant3/1 -> Vitis HLS1/1
  Vitis HLS1/1 -> Terminator/1
  Vitis HLS1/2 -> Terminator1/1
  Vitis HLS1/3 -> Terminator2/1
  Vitis HLS1/4 -> Terminator3/1
  Vitis HLS1/5 -> Terminator4/1
  Vitis HLS1/6 -> Terminator5/1
  Vitis HLS1/11 -> Terminator7/1
  Register/1 -> Mux/3, Vitis HLS1/3
  Vitis HLS1/8 -> Register/2
  Vitis HLS1/7 -> Register/1
  Constant11/1 -> Mux4/2
  Mux4/1 -> Out9/1
  Vitis HLS1/9 -> Mux4/3
  Vitis HLS1/10 -> Mux4/1
  In1/1 -> Delay1/1, Mux/1
  Constant1/1 -> Mux/2
  Mux/1 -> Negate1/1
  Negate1/1 -> Gateway Out/1
  Gateway Out/1 -> To Workspace12/1
  Delay1/1 -> Out2/1, Out4/1
  Vitis HLS1/12 -> Terminator16/1

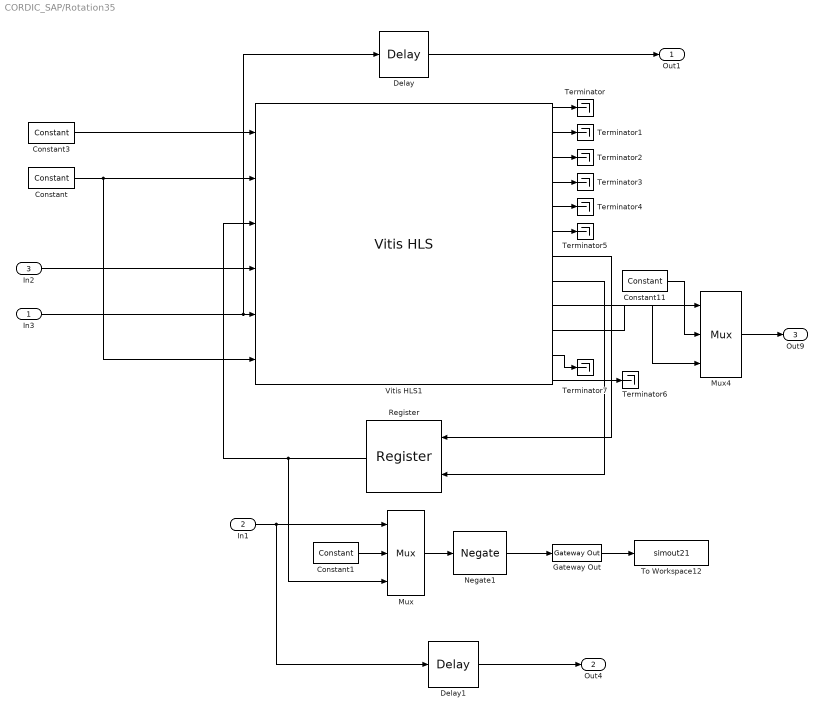
== system CORDIC_SAP/Rotation35 ==
  In3 : Inport
  In1 : Inport  Port=2
  In2 : Inport  Port=3
  Constant : hdlBasic/Constant  const=1.0  gui_display_data_type=Boolean  arith_type=Boolean  n_bits=16  bin_pt=14  preci_type=Single  exp_width=8  frac_width=24  explicit_period=off  period=1  XmcBlockStatus=1  maskContainerNames=tabcontainer1  block_type=constant  block_config=sysgen:Constant_config
  Constant1 : hdlBasic/Constant  const=0  gui_display_data_type=Fixed-point  arith_type=Signed (2's comp)  n_bits=16  bin_pt=13  preci_type=Single  exp_width=8  frac_width=24  explicit_period=off  period=1  XmcBlockStatus=1  maskContainerNames=tabcontainer1  block_type=constant  block_config=sysgen:Constant_config
  Constant11 : hdlBasic/Constant  const=0  gui_display_data_type=Fixed-point  arith_type=Signed (2's comp)  n_bits=16  bin_pt=13  preci_type=Single  exp_width=8  frac_width=24  explicit_period=off  period=1  XmcBlockStatus=1  maskContainerNames=tabcontainer1  block_type=constant  block_config=sysgen:Constant_config
  Constant3 : hdlBasic/Constant  const=0  gui_display_data_type=Boolean  arith_type=Boolean  n_bits=16  bin_pt=14  preci_type=Single  exp_width=8  frac_width=24  explicit_period=off  period=1  XmcBlockStatus=1  maskContainerNames=tabcontainer1  block_type=constant  block_config=sysgen:Constant_config
  Delay : hdlBasic/Delay  rst=off  en=off  latency=27  reg_retiming=off  XmcBlockStatus=1  maskContainerNames=group1  block_type=delay  block_config=sysgen:Delay_config
  Delay1 : hdlBasic/Delay  rst=off  en=off  latency=27  reg_retiming=off  XmcBlockStatus=1  maskContainerNames=group1  block_type=delay  block_config=sysgen:Delay_config
  Gateway Out : hdlBasic/Gateway Out  inherit_from_input=off  hdl_port=on  rows=1  columns=1  UseAsDAC=off  DACChannel='1'  interface=AXI4-Lite  automatic_assignment=on  address_offset=hex2dec('00')  intf_name=''  intf_description='R_1_3'  timing_constraint=None  locs_specified=off  LOCs={}  io_standard={}  XmcBlockStatus=1  maskContainerNames=group4  block_type=gatewayout  block_config=sysgen:gateway_out_config  block_width_w=590  block_height_w=620  block_width=620  block_height=750
  Mux : hdlBasic/Mux  inputs=2  en=off  latency=1  precision=Full  arith_type=Unsigned  n_bits=16  bin_pt=14  quantization=Truncate  overflow=Wrap  XmcBlockStatus=1  maskContainerNames=tabcontainer1  block_type=mux  block_config=sysgen:Mux_config
  Mux4 : hdlBasic/Mux  inputs=2  en=off  latency=1  precision=Full  arith_type=Unsigned  n_bits=16  bin_pt=14  quantization=Truncate  overflow=Wrap  XmcBlockStatus=1  maskContainerNames=tabcontainer1  block_type=mux  block_config=sysgen:Mux_config
  Negate1 : hdlBasic/Negate  precision=Full  arith_type=Unsigned  n_bits=16  bin_pt=14  quantization=Truncate  overflow=Wrap  en=off  latency=0  XmcBlockStatus=1  maskContainerNames=tabcontainer1  block_type=negate  block_config=sysgen:Negate_config
  Register : hdlBasic/Register  init=0  rst=off  en=on  XmcBlockStatus=1  maskContainerNames=tabcontainer1  block_type=register  block_config=sysgen:Register_config
  Terminator{,1..7} (8 alike) : Terminator
  To Workspace12 : ToWorkspace  VariableName=simout21  SaveFormat=Timeseries  SampleTime=-1
  Vitis HLS1 : hdlBasic/Vitis HLS  anytable='C:\ELEC522\jz118\HLS\cordic\solution1'  fast_sim=off  display_datatype=off  rate_propagation_method=Simulink system period  model_file_path=''  latency=1  block_type=vitis_hls
      settings: infoedit=This block allows including C,C++ and SystemC source files in System Generator for DSP designs.
  Out1 : Outport
  Out4 : Outport  Port=2
  Out9 : Outport  Port=3
  wires:
  In2/1 -> Vitis HLS1/4
  In3/1 -> Delay/1, Vitis HLS1/5
  Delay/1 -> Out1/1
  Constant/1 -> Vitis HLS1/2, Vitis HLS1/6
  Constant3/1 -> Vitis HLS1/1
  Vitis HLS1/1 -> Terminator/1
  Vitis HLS1/2 -> Terminator1/1
  Vitis HLS1/3 -> Terminator2/1
  Vitis HLS1/4 -> Terminator3/1
  Vitis HLS1/5 -> Terminator4/1
  Vitis HLS1/6 -> Terminator5/1
  Vitis HLS1/11 -> Terminator7/1
  Register/1 -> Mux/3, Vitis HLS1/3
  Vitis HLS1/8 -> Register/2
  Vitis HLS1/7 -> Register/1
  Constant11/1 -> Mux4/2
  Mux4/1 -> Out9/1
  Vitis HLS1/9 -> Mux4/3
  Vitis HLS1/10 -> Mux4/1
  In1/1 -> Delay1/1, Mux/1
  Constant1/1 -> Mux/2
  Mux/1 -> Negate1/1
  Negate1/1 -> Gateway Out/1
  Gateway Out/1 -> To Workspace12/1
  Delay1/1 -> Out4/1
  Vitis HLS1/12 -> Terminator6/1

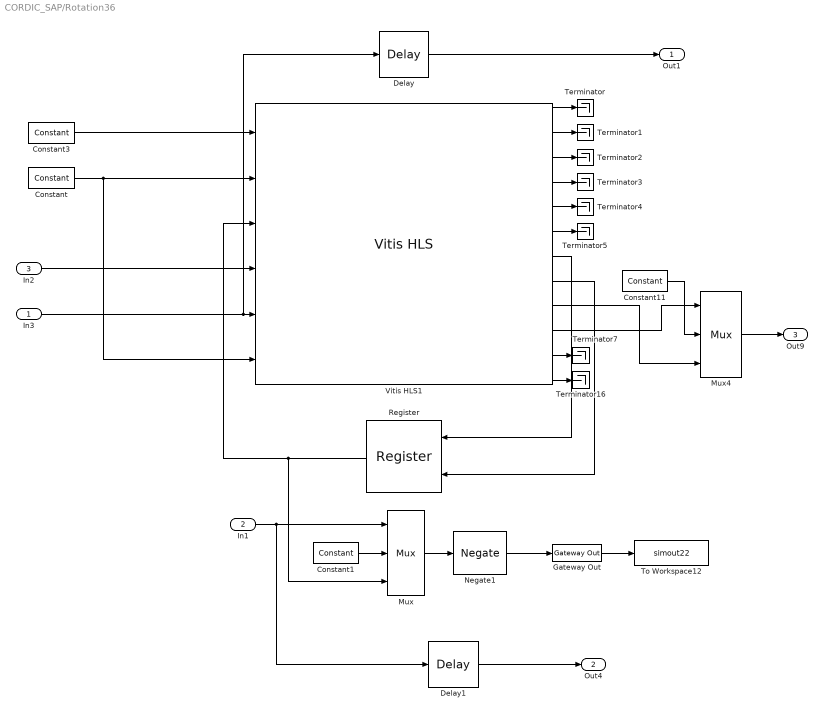
== system CORDIC_SAP/Rotation36 ==
  In3 : Inport
  In1 : Inport  Port=2
  In2 : Inport  Port=3
  Constant : hdlBasic/Constant  const=1.0  gui_display_data_type=Boolean  arith_type=Boolean  n_bits=16  bin_pt=14  preci_type=Single  exp_width=8  frac_width=24  explicit_period=off  period=1  XmcBlockStatus=1  maskContainerNames=tabcontainer1  block_type=constant  block_config=sysgen:Constant_config
  Constant1 : hdlBasic/Constant  const=0  gui_display_data_type=Fixed-point  arith_type=Signed (2's comp)  n_bits=16  bin_pt=13  preci_type=Single  exp_width=8  frac_width=24  explicit_period=off  period=1  XmcBlockStatus=1  maskContainerNames=tabcontainer1  block_type=constant  block_config=sysgen:Constant_config
  Constant11 : hdlBasic/Constant  const=0  gui_display_data_type=Fixed-point  arith_type=Signed (2's comp)  n_bits=16  bin_pt=13  preci_type=Single  exp_width=8  frac_width=24  explicit_period=off  period=1  XmcBlockStatus=1  maskContainerNames=tabcontainer1  block_type=constant  block_config=sysgen:Constant_config
  Constant3 : hdlBasic/Constant  const=0  gui_display_data_type=Boolean  arith_type=Boolean  n_bits=16  bin_pt=14  preci_type=Single  exp_width=8  frac_width=24  explicit_period=off  period=1  XmcBlockStatus=1  maskContainerNames=tabcontainer1  block_type=constant  block_config=sysgen:Constant_config
  Delay : hdlBasic/Delay  rst=off  en=off  latency=27  reg_retiming=off  XmcBlockStatus=1  maskContainerNames=group1  block_type=delay  block_config=sysgen:Delay_config
  Delay1 : hdlBasic/Delay  rst=off  en=off  latency=27  reg_retiming=off  XmcBlockStatus=1  maskContainerNames=group1  block_type=delay  block_config=sysgen:Delay_config
  Gateway Out : hdlBasic/Gateway Out  inherit_from_input=off  hdl_port=on  rows=1  columns=1  UseAsDAC=off  DACChannel='1'  interface=AXI4-Lite  automatic_assignment=on  address_offset=hex2dec('00')  intf_name=''  intf_description='R_1_4'  timing_constraint=None  locs_specified=off  LOCs={}  io_standard={}  XmcBlockStatus=1  maskContainerNames=group4  block_type=gatewayout  block_config=sysgen:gateway_out_config  block_width_w=590  block_height_w=620  block_width=620  block_height=750
  Mux : hdlBasic/Mux  inputs=2  en=off  latency=1  precision=Full  arith_type=Unsigned  n_bits=16  bin_pt=14  quantization=Truncate  overflow=Wrap  XmcBlockStatus=1  maskContainerNames=tabcontainer1  block_type=mux  block_config=sysgen:Mux_config
  Mux4 : hdlBasic/Mux  inputs=2  en=off  latency=1  precision=Full  arith_type=Unsigned  n_bits=16  bin_pt=14  quantization=Truncate  overflow=Wrap  XmcBlockStatus=1  maskContainerNames=tabcontainer1  block_type=mux  block_config=sysgen:Mux_config
  Negate1 : hdlBasic/Negate  precision=Full  arith_type=Unsigned  n_bits=16  bin_pt=14  quantization=Truncate  overflow=Wrap  en=off  latency=0  XmcBlockStatus=1  maskContainerNames=tabcontainer1  block_type=negate  block_config=sysgen:Negate_config
  Register : hdlBasic/Register  init=0  rst=off  en=on  XmcBlockStatus=1  maskContainerNames=tabcontainer1  block_type=register  block_config=sysgen:Register_config
  Terminator{,1..5,7,16} (8 alike) : Terminator
  To Workspace12 : ToWorkspace  VariableName=simout22  SaveFormat=Timeseries  SampleTime=-1
  Vitis HLS1 : hdlBasic/Vitis HLS  anytable='C:\ELEC522\jz118\HLS\cordic\solution1'  fast_sim=off  display_datatype=off  rate_propagation_method=Simulink system period  model_file_path=''  latency=1  block_type=vitis_hls
      settings: infoedit=This block allows including C,C++ and SystemC source files in System Generator for DSP designs.
  Out1 : Outport
  Out4 : Outport  Port=2
  Out9 : Outport  Port=3
  wires:
  In2/1 -> Vitis HLS1/4
  In3/1 -> Delay/1, Vitis HLS1/5
  Delay/1 -> Out1/1
  Constant/1 -> Vitis HLS1/2, Vitis HLS1/6
  Constant3/1 -> Vitis HLS1/1
  Vitis HLS1/1 -> Terminator/1
  Vitis HLS1/2 -> Terminator1/1
  Vitis HLS1/3 -> Terminator2/1
  Vitis HLS1/4 -> Terminator3/1
  Vitis HLS1/5 -> Terminator4/1
  Vitis HLS1/6 -> Terminator5/1
  Vitis HLS1/11 -> Terminator7/1
  Vitis HLS1/12 -> Terminator16/1
  Register/1 -> Mux/3, Vitis HLS1/3
  Vitis HLS1/8 -> Register/2
  Vitis HLS1/7 -> Register/1
  Constant11/1 -> Mux4/2
  Mux4/1 -> Out9/1
  Vitis HLS1/9 -> Mux4/3
  Vitis HLS1/10 -> Mux4/1
  In1/1 -> Delay1/1, Mux/1
  Constant1/1 -> Mux/2
  Mux/1 -> Negate1/1
  Negate1/1 -> Gateway Out/1
  Gateway Out/1 -> To Workspace12/1
  Delay1/1 -> Out4/1
